simulink model "pmsm_vector_ctrl_osm_2021_07_20"  (R2020a)
settings: Solver=daessc  StartTime=0.0  StopTime=simlength  MaxStep=Ts/10
values from neighbouring files (symbols this model uses):
  dead_time = 0    [init_pmsm_2021_07_20_newDesign.m]    (also in init_pmsm_2021_07_20_oldDesign.m)
  delayINV_modA = 0    [init_pmsm_2021_07_20_newDesign.m]    (also in init_pmsm_2021_07_20_oldDesign.m)
  fPWM_INV = 8e3    (= 8000)    [init_pmsm_2021_07_20_newDesign.m]    (also in init_pmsm_2021_07_20_oldDesign.m)
  Ibez = 550    [init_pmsm_2021_07_20_newDesign.m]    (also in init_pmsm_2021_07_20_oldDesign.m)
  Jm = 1    [init_pmsm_2021_07_20_newDesign.m]    (also in init_pmsm_2021_07_20_oldDesign.m)
  ki = 18    [init_pmsm_2021_07_20_newDesign.m]    (also in init_pmsm_2021_07_20_oldDesign.m)
  kp = 2    [init_pmsm_2021_07_20_newDesign.m]    (also in init_pmsm_2021_07_20_oldDesign.m)
  Ld = 2.77e-3    (= 0.00277)    [init_pmsm_2021_07_20_newDesign.m]    (also in init_pmsm_2021_07_20_oldDesign.m = 0.00267)
  Lq = 3.77e-3    (= 0.00377)    [init_pmsm_2021_07_20_newDesign.m]    (also in init_pmsm_2021_07_20_oldDesign.m = 0.00328)
  number_poles = 8    [init_pmsm_2021_07_20_newDesign.m]    (also in init_pmsm_2021_07_20_oldDesign.m)
  psi_m = 0.5    [init_pmsm_2021_07_20_newDesign.m]    (also in init_pmsm_2021_07_20_oldDesign.m = 0.37)
  simlength = 5    [init_pmsm_2021_07_20_newDesign.m]    (also in init_pmsm_2021_07_20_oldDesign.m)
  Tc = 1e-5    (= 1e-05)    [init_pmsm_2021_07_20_newDesign.m]    (also in init_pmsm_2021_07_20_oldDesign.m)
  Ts = tPWM_INV/2    (= 3.125e-05)    [init_pmsm_2021_07_20_newDesign.m]    (also in init_pmsm_2021_07_20_oldDesign.m)
libraries: nesl_utility x25, fl_lib x23, ee_lib x6, flexshaft_lib x1, pmsm_uvw_lib x1
(part 1 of 2)
settings Model: SimulationMode=accelerator  Creator=dbagn  LastModifiedBy=dbagn
settings SolverCC: ZeroCrossControl=DisableAll  SolverResetMethod=Robust
settings DataIOCC: ReturnWorkspaceOutputs=off

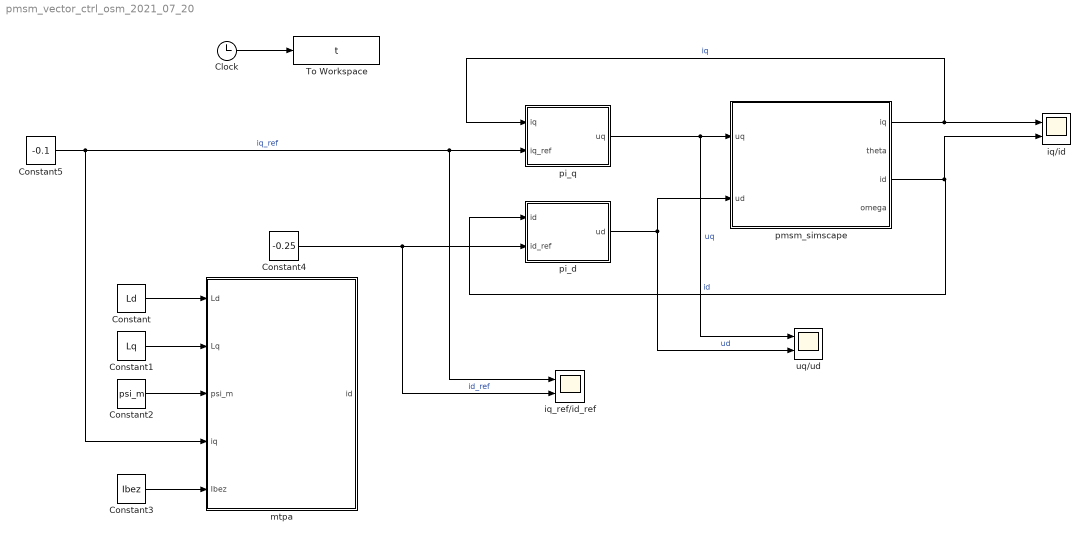
== system pmsm_vector_ctrl_osm_2021_07_20 ==
  Clock : Clock
  Constant : Constant  Value=Ld
  Constant1 : Constant  Value=Lq
  Constant2 : Constant  Value=psi_m
  Constant3 : Constant  Value=Ibez
  Constant4 : Constant  Value=-0.25
  Constant5 : Constant  Value=-0.1
  To Workspace : ToWorkspace  VariableName=t  SampleTime=Tc
      settings: MaxDataPoints=Nc
  iq/id : Scope  NumInputPorts=2
  iq_ref/id_ref : Scope  NumInputPorts=2
  mtpa : MATLAB Function  TreatAsAtomicUnit=on  SystemSampleTime=Ts
  pi_d : Subsystem  mask{kp=kp, ki=ki, ts=Ts, sat_pos=sqrt(3)/2, sat_neg=-sqrt(3)/2}
  pi_q : Subsystem  mask{kp=kp, ki=ki, ts=Ts, sat_pos=sqrt(3)/2, sat_neg=-sqrt(3)/2}
  pmsm_simscape : Subsystem
  uq/ud : Scope  NumInputPorts=2
  wires:
  Clock/1 -> To Workspace/1
  Constant5/1 -> pi_q/2(iq_ref), iq_ref/id_ref/1, mtpa/4(iq)  "iq_ref"
  pmsm_simscape/1(iq) -> iq/id/1, pi_q/1(iq)  "iq"
  pi_q/1(uq) -> uq/ud/1, pmsm_simscape/1(uq)  "uq"
  pi_d/1(ud) -> uq/ud/2, pmsm_simscape/2(ud)  "ud"
  pmsm_simscape/3(id) -> iq/id/2, pi_d/1(id)  "id"
  Constant2/1 -> mtpa/3(psi_m)
  Constant1/1 -> mtpa/2(Lq)
  Constant/1 -> mtpa/1(Ld)
  Constant3/1 -> mtpa/5(Ibez)
  Constant4/1 -> iq_ref/id_ref/2, pi_d/2(id_ref)  "id_ref"

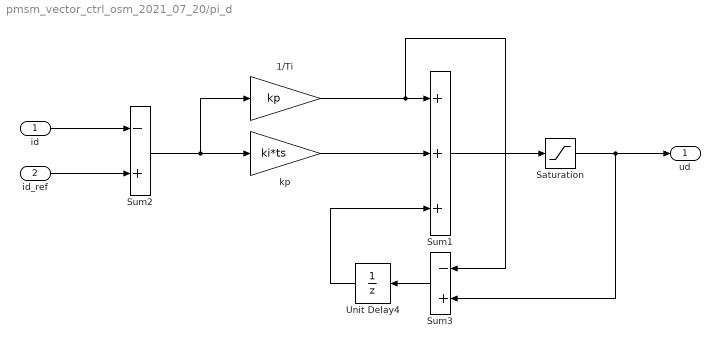
== system pmsm_vector_ctrl_osm_2021_07_20/pi_d ==
  id : Inport
  id_ref : Inport  Port=2
  1/Ti : Gain  Gain=kp  SaturateOnIntegerOverflow=on  OutDataTypeStr=Inherit: Same as input  ParamDataTypeStr=Inherit: Same as input
  Saturation : Saturate  UpperLimit=sat_pos  LowerLimit=sat_neg
  Sum1 : Sum  Inputs=+++  SaturateOnIntegerOverflow=on
  Sum2 : Sum  Inputs=-+  SaturateOnIntegerOverflow=on
  Sum3 : Sum  Inputs=-+  SaturateOnIntegerOverflow=on
  Unit Delay4 : UnitDelay  SampleTime=ts  HasFrameUpgradeWarning=on
  kp : Gain  Gain=ki*ts  SaturateOnIntegerOverflow=on  OutDataTypeStr=Inherit: Same as input  ParamDataTypeStr=Inherit: Same as input
  ud : Outport
  wires:
  Saturation/1 -> Sum3/2, ud/1
  Unit Delay4/1 -> Sum1/3
  Sum1/1 -> Saturation/1
  id/1 -> Sum2/1
  Sum3/1 -> Unit Delay4/1
  1/Ti/1 -> Sum3/1, Sum1/1
  Sum2/1 -> 1/Ti/1, kp/1
  kp/1 -> Sum1/2
  id_ref/1 -> Sum2/2

== system pmsm_vector_ctrl_osm_2021_07_20/pi_q ==
  iq : Inport
  iq_ref : Inport  Port=2
  1/Ti : Gain  Gain=kp  SaturateOnIntegerOverflow=on  OutDataTypeStr=Inherit: Same as input  ParamDataTypeStr=Inherit: Same as input
  Saturation : Saturate  UpperLimit=sat_pos  LowerLimit=sat_neg
  Sum1 : Sum  Inputs=+++  SaturateOnIntegerOverflow=on
  Sum2 : Sum  Inputs=-+  SaturateOnIntegerOverflow=on
  Sum3 : Sum  Inputs=-+  SaturateOnIntegerOverflow=on
  Unit Delay4 : UnitDelay  SampleTime=ts  HasFrameUpgradeWarning=on
  kp : Gain  Gain=ki*ts  SaturateOnIntegerOverflow=on  OutDataTypeStr=Inherit: Same as input  ParamDataTypeStr=Inherit: Same as input
  uq : Outport
  wires:
  iq_ref/1 -> Sum2/2
  kp/1 -> Sum1/2
  Sum2/1 -> kp/1, 1/Ti/1
  1/Ti/1 -> Sum1/1, Sum3/1
  Sum3/1 -> Unit Delay4/1
  iq/1 -> Sum2/1
  Sum1/1 -> Saturation/1
  Unit Delay4/1 -> Sum1/3
  Saturation/1 -> uq/1, Sum3/2

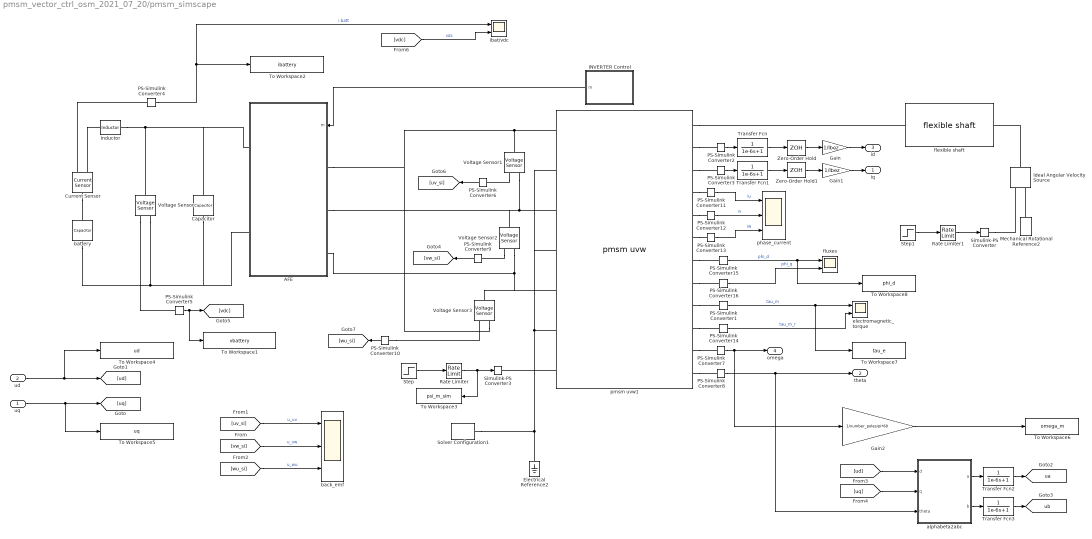
== system pmsm_vector_ctrl_osm_2021_07_20/pmsm_simscape ==
  uq : Inport
  ud : Inport  Port=2
  AFE : Subsystem
  Capacitor : fl_lib/Electrical/Electrical Elements/Capacitor  c=5e-3 F  r=1e-3 Ohm  g=0 1/Ohm  i_specify=off  i_priority=None  i=0 A  i_nominal_specify=off  i_nominal_unit=A  i_nominal_value=1  v_specify=off  v_priority=High  v=350 V  v_nominal_specify=off  v_nominal_unit=V  v_nominal_value=1  vc_specify=on  vc_priority=High  vc=Vdc V  vc_nominal_specify=off  vc_nominal_unit=V  vc_nominal_value=1
  Current Sensor : fl_lib/Electrical/Electrical Sensors/Current Sensor
  Electrical Reference2 : fl_lib/Electrical/Electrical Elements/Electrical Reference
  Gain : Gain  Gain=1/Ibez
  Gain1 : Gain  Gain=1/Ibez
  Gain2 : Gain  Gain=1/number_poles/pi*60
  INVERTER Control : Subsystem
  Ideal Angular Velocity Source : fl_lib/Mechanical/Mechanical Sources/Ideal Angular Velocity Source
  Inductor : fl_lib/Electrical/Electrical Elements/Inductor  l=20e-6 H  r=1e-3 Ohm  g=1e-9 1/Ohm  i_specify=off  i_priority=None  i=0 A  i_nominal_specify=off  i_nominal_unit=A  i_nominal_value=1  v_specify=off  v_priority=None  v=0 V  v_nominal_specify=off  v_nominal_unit=V  v_nominal_value=1  i_L_specify=off  i_L_priority=High  i_L=0 A  i_L_nominal_specify=off  i_L_nominal_unit=A  i_L_nominal_value=1
  Mechanical Rotational Reference2 : fl_lib/Mechanical/Rotational Elements/Mechanical Rotational Reference
  PS-Simulink Converter1 : nesl_utility/PS-Simulink Converter  PhysicalDomain=network_engine_domain  SubClassName=ps_output  LeftPortType=input  RightPortType=output  PseudoPeriodic=off  Frequencies=[]  Unit=N*m  AffineConversion=on
  PS-Simulink Converter{2..4,6,9..10} (6 alike) : nesl_utility/PS-Simulink Converter  PhysicalDomain=network_engine_domain  SubClassName=ps_output  LeftPortType=input  RightPortType=output  PseudoPeriodic=off  Frequencies=[]  Unit=1  AffineConversion=off
  PS-Simulink Converter11 : nesl_utility/PS-Simulink Converter  PhysicalDomain=network_engine_domain  SubClassName=ps_output  LeftPortType=input  RightPortType=output  PseudoPeriodic=off  Frequencies=[]  Unit=A  AffineConversion=on
  PS-Simulink Converter12 : nesl_utility/PS-Simulink Converter  PhysicalDomain=network_engine_domain  SubClassName=ps_output  LeftPortType=input  RightPortType=output  PseudoPeriodic=off  Frequencies=[]  Unit=A  AffineConversion=on
  PS-Simulink Converter13 : nesl_utility/PS-Simulink Converter  PhysicalDomain=network_engine_domain  SubClassName=ps_output  LeftPortType=input  RightPortType=output  PseudoPeriodic=off  Frequencies=[]  Unit=A  AffineConversion=on
  PS-Simulink Converter14 : nesl_utility/PS-Simulink Converter  PhysicalDomain=network_engine_domain  SubClassName=ps_output  LeftPortType=input  RightPortType=output  PseudoPeriodic=off  Frequencies=[]  Unit=N*m  AffineConversion=on
  PS-Simulink Converter15 : nesl_utility/PS-Simulink Converter  PhysicalDomain=network_engine_domain  SubClassName=ps_output  LeftPortType=input  RightPortType=output  PseudoPeriodic=off  Frequencies=[]  Unit=V*s  AffineConversion=on
  PS-Simulink Converter16 : nesl_utility/PS-Simulink Converter  PhysicalDomain=network_engine_domain  SubClassName=ps_output  LeftPortType=input  RightPortType=output  PseudoPeriodic=off  Frequencies=[]  Unit=V*s  AffineConversion=on
  PS-Simulink Converter5 : nesl_utility/PS-Simulink Converter  PhysicalDomain=network_engine_domain  SubClassName=ps_output  LeftPortType=input  RightPortType=output  PseudoPeriodic=off  Frequencies=[]  Unit=V  AffineConversion=on
  PS-Simulink Converter7 : nesl_utility/PS-Simulink Converter  PhysicalDomain=network_engine_domain  SubClassName=ps_output  LeftPortType=input  RightPortType=output  PseudoPeriodic=off  Frequencies=[]  Unit=rad/s  AffineConversion=on
  PS-Simulink Converter8 : nesl_utility/PS-Simulink Converter  PhysicalDomain=network_engine_domain  SubClassName=ps_output  LeftPortType=input  RightPortType=output  PseudoPeriodic=off  Frequencies=[]  Unit=rad  AffineConversion=on
  Rate Limiter : RateLimiter  RisingSlewLimit=0.1  FallingSlewLimit=-0.1  SampleTimeMode=inherited
  Rate Limiter1 : RateLimiter  RisingSlewLimit=3100/2  FallingSlewLimit=-3100/2  SampleTimeMode=inherited
  Simulink-PS Converter : nesl_utility/Simulink-PS Converter  PhysicalDomain=network_engine_domain  SubClassName=ps_input  LeftPortType=input  RightPortType=output  PseudoPeriodic=off  Frequencies=[]  NoiseDistribution=none  NoiseParameters=[]  Unit=rpm  AffineConversion=on  FilteringAndDerivatives=provide  SimscapeFilterOrder=1  InputFilterTimeConstant=0.001  UdotUserProvided=0
  Simulink-PS Converter3 : nesl_utility/Simulink-PS Converter  PhysicalDomain=network_engine_domain  SubClassName=ps_input  LeftPortType=input  RightPortType=output  PseudoPeriodic=off  Frequencies=[]  NoiseDistribution=none  NoiseParameters=[]  Unit=V*s  AffineConversion=off  FilteringAndDerivatives=provide  SimscapeFilterOrder=1  InputFilterTimeConstant=0.001  UdotUserProvided=0
  Solver Configuration1 : nesl_utility/Solver Configuration  PhysicalDomain=network_engine_domain  SubClassName=solver  LeftPortType=input  RightPortType=generic  Tones=[]  Harmonics=[]  SimulateNoise=off  Profile=off  UseLocalSampling=off  EnableSwitchedLinearOptims=on  FrequencyDomain=off  UseCCode=off  RelTol=0.001  AbsTol=1e-06  MinStep=1e-09  ToWorkspace=off  RevertToSquareIcSolve=off  NumHomotopyIterations=100  PhasorMode=off  PhasorModeNumHarmonics=1  DoDC=off  ResidualTolerance=1e-09  UseLocalSolver=on  LocalSolverChoice=NE_BACKWARD_EULER_ADVANCER  LocalSolverSampleTime=Ts/10  DoFixedCost=on  MaxNonlinIter=3  MaxModeIter=2  LinearAlgebra=auto  EquationFormulation=NE_TIME_EF  DelaysMemoryBudget=1024*4  AutomaticFiltering=on  FilteringTimeConstant=Ts  PartitionStorageMethod=AS_NEEDED  PartitionMemoryBudget=1024  PartitionMethod=ROBUST
  Step : Step  Time=simlength/2  Before=psi_m  After=psi_m  SampleTime=0
  Step1 : Step  Time=1e-2  After=3100  SampleTime=0
  To Workspace1 : ToWorkspace  VariableName=vbattery  SampleTime=Tc
      settings: MaxDataPoints=Nc
  To Workspace2 : ToWorkspace  VariableName=ibattery  SampleTime=Tc
      settings: MaxDataPoints=Nc
  To Workspace3 : ToWorkspace  VariableName=psi_m_sim  SampleTime=Tc
      settings: MaxDataPoints=Nc
  To Workspace4 : ToWorkspace  VariableName=ud  SampleTime=Tc
      settings: MaxDataPoints=Nc
  To Workspace5 : ToWorkspace  VariableName=uq  SampleTime=Tc
      settings: MaxDataPoints=Nc
  To Workspace6 : ToWorkspace  VariableName=omega_m  SampleTime=Tc
      settings: MaxDataPoints=Nc
  To Workspace7 : ToWorkspace  VariableName=tau_e  SampleTime=Tc
      settings: MaxDataPoints=Nc
  To Workspace8 : ToWorkspace  VariableName=phi_d  SampleTime=Tc
      settings: MaxDataPoints=Nc
  Transfer Fcn{,1..3} (4 alike) : TransferFcn  Denominator=[1e-6 1]
  Voltage Sensor{,1..3} (4 alike) : fl_lib/Electrical/Electrical Sensors/Voltage Sensor
  Zero-Order Hold : ZeroOrderHold  SampleTime=Ts
  Zero-Order Hold1 : ZeroOrderHold  SampleTime=Ts
  alphabeta2abc : Subsystem
  back_emf : Scope  NumInputPorts=3
  battery : fl_lib/Electrical/Electrical Elements/Capacitor  c=1500 F  r=0.05 Ohm  g=0 1/Ohm  i_specify=off  i_priority=None  i=0 A  i_nominal_specify=off  i_nominal_unit=A  i_nominal_value=1  v_specify=off  v_priority=High  v=350 V  v_nominal_specify=off  v_nominal_unit=V  v_nominal_value=1  vc_specify=on  vc_priority=High  vc=Vdc V  vc_nominal_specify=off  vc_nominal_unit=V  vc_nominal_value=1
  electromagnetic_torque : Scope  NumInputPorts=2
  flexible shaft : flexshaft_lib/flexible shaft  b1=0 N*m/(rad/s)  J1=0.125 kg*m^2  b2=0 N*m/(rad/s)  J2=0.125 kg*m^2  b_theta=1 N*m/(rad/s)  k_theta=1e5 N*m/rad  w_1_specify=off  w_1_priority=None  w_1=0 rad/s  w_1_nominal_specify=off  w_1_nominal_unit=rad/s  w_1_nominal_value=1  w_2_specify=off  w_2_priority=None  w_2=0 rad/s  w_2_nominal_specify=off  w_2_nominal_unit=rad/s  w_2_nominal_value=1  t_1_specify=off  t_1_priority=None  t_1=0 N*m  t_1_nominal_specify=off  t_1_nominal_unit=N*m  t_1_nominal_value=1  t_2_specify=off  t_2_priority=None  t_2=0 N*m  t_2_nominal_specify=off  t_2_nominal_unit=N*m  t_2_nominal_value=1  t_theta_specify=off  t_theta_priority=None  t_theta=0 N*m  t_theta_nominal_specify=off  t_theta_nominal_unit=N*m  t_theta_nominal_value=1
      settings: InternalSimscapePortConfiguration="{\"Bottom\":[],\"Left\":[{\"id\":\"S1\",\"label\":\"S1\",\"type\":\"foundation.mechanical.rotational.rotational\"}],\"Right\":[{\"id\":\"S2\",\"label\":\"S2\",\"type\":\"foundation.mechanical.rotational.rotational\"}],\"Top\":[]}"
  fluxes : Scope  NumInputPorts=2
  ibat/vdc : Scope  NumInputPorts=2
  phase_current : Scope  NumInputPorts=3
  pmsm uvw1 : pmsm_uvw_lib/pmsm uvw  number_poles=number_poles  psi_M=psi_m s*V  Lmu=Lmu H  Ls=Ls H  Lb=Lb H  Rs=Rs Ohm  J=Jm kg*m^2  b=0 N*m/(rad/s)  omega_specify=off  omega_priority=None  omega=0 rad/s  omega_nominal_specify=off  omega_nominal_unit=rad/s  omega_nominal_value=1  theta_specify=off  theta_priority=None  theta=0 rad  theta_nominal_specify=off  theta_nominal_unit=rad  theta_nominal_value=1  iu_specify=off  iu_priority=None  iu=0 A  iu_nominal_specify=off  iu_nominal_unit=A  iu_nominal_value=1  iv_specify=off  iv_priority=None  iv=0 A  iv_nominal_specify=off  iv_nominal_unit=A  iv_nominal_value=1  iw_specify=off  iw_priority=None  iw=0 A  iw_nominal_specify=off  iw_nominal_unit=A  iw_nominal_value=1  id_specify=off  id_priority=None  id=0 A  id_nominal_specify=off  id_nominal_unit=A  id_nominal_value=1  iq_specify=off  iq_priority=None  iq=0 A  iq_nominal_specify=off  iq_nominal_unit=A  iq_nominal_value=1  uv_specify=off  uv_priority=None  uv=0 V  uv_nominal_specify=off  uv_nominal_unit=V  uv_nominal_value=1  uu_specify=off  uu_priority=None  uu=0 V  uu_nominal_specify=off  uu_nominal_unit=V  uu_nominal_value=1  uw_specify=off  uw_priority=None  uw=0 V  uw_nominal_specify=off  uw_nominal_unit=V  uw_nominal_value=1  phi_u_specify=on  phi_u_priority=High  phi_u=psi_m s*V  phi_u_nominal_specify=off  phi_u_nominal_unit=s*V  phi_u_nominal_value=1  phi_v_specify=on  phi_v_priority=High  phi_v=-psi_m/2 s*V  phi_v_nominal_specify=off  phi_v_nominal_unit=s*V  phi_v_nominal_value=1  phi_w_specify=on  phi_w_priority=High  phi_w=-psi_m/2 s*V  phi_w_nominal_specify=off  phi_w_nominal_unit=s*V  phi_w_nominal_value=1  phi_d_specify=off  phi_d_priority=None  phi_d=psi_m s*V  phi_d_nominal_specify=off  phi_d_nominal_unit=s*V  phi_d_nominal_value=1  phi_q_specify=off  phi_q_priority=None  phi_q=0 s*V  phi_q_nominal_specify=off  phi_q_nominal_unit=s*V  phi_q_nominal_value=1  psi_d_specify=off  psi_d_priority=None  psi_d=0 s*V  psi_d_nominal_specify=off  psi_d_nominal_unit=s*V  psi_d_nominal_value=1  psi_q_specify=off  psi_q_priority=None  psi_q=0 s*V  psi_q_nominal_specify=off  psi_q_nominal_unit=s*V  psi_q_nominal_value=1  tau_l_specify=off  tau_l_priority=None  tau_l=0 N*m  tau_l_nominal_specify=off  tau_l_nominal_unit=N*m  tau_l_nominal_value=1  tau_m_specify=off  tau_m_priority=None  tau_m=0 N*m  tau_m_nominal_specify=off  tau_m_nominal_unit=N*m  tau_m_nominal_value=1  tau_m_r_specify=off  tau_m_r_priority=None  tau_m_r=0 N*m  tau_m_r_nominal_specify=off  tau_m_r_nominal_unit=N*m  tau_m_r_nominal_value=1
      settings: InternalSimscapePortConfiguration="{\"Bottom\":[],\"Left\":[{\"id\":\"uu_p\",\"label\":\"_uu+_\",\"type\":\"foundation.electrical.electrical\"},{\"id\":\"uu_n\",\"label\":\"_uu-_\",\"type\":\"foundation.electrical.electrical\"},{\"id\":\"uv_p\",\"label\":\"_uv+_\",\"type\":\"foundation.electrical.electrical\"},{\"id\":\"uv_n\",\"label\":\"_uv-_\",\"type\":\"foundation.electrical.electrical\"},{\"id\":\"uw_p\",\"label\":\"_uw+_\",\"type\":\"foundation.electrical.electrical\"},{\"id\":\"uw_n\",\"label\":\"_uw-_\",\"type\":\"foundation.electrical.electrical\"},{\"id\":\"psi_m\",\"label\":\"_psi_m_\",\"type\":\"input\"}],\"Right\":[{\"id\":\"S\",\"label\":\"_S_\",\"type\":\"foundation.mechanical.rotational.rotational\"},{\"id\":\"id_out\",\"label\":\"_id_\",\"type\":\"output\"},{\"id\":\"iq_out\",\"label\":\"_iq_\",\"type\":\"output\"},{\"id\":\"iu_out\",\"label\":\"_iu_\",\"type\":\"output\"},{\"id\":\"iv_out\",\"label\":\"_iv_\",\"type\":\"output\"},{\"id\":\"iw_out\",\"label\":\"_iw_\",\"type\":\"output\"},{\"id\":\"phi_d_out\",\"label\":\"_phi_d_\",\"type\":\"output\"},{\"id\":\"phi_q_out\",\"label\":\"_phi_q\",\"type\":\"output\"},{\"id\":\"tau_out\",\"label\":\"_torque_\",\"type\":\"output\"},{\"id\":\"tau_out_r\",\"label\":\"_torque_r_\",\"type\":\"output\"},{\"id\":\"omega_out\",\"label\":\"_omega_elec_\",\"type\":\"output\"},{\"id\":\"theta_out\",\"label\":\"_theta_elec_\",\"type\":\"output\"}],\"Top\":[]}"
  iq : Outport
  theta : Outport  Port=2
  id : Outport  Port=3
  omega : Outport  Port=4
  tag scope: ua=global, ub=global
  wires:
  PS-Simulink Converter2/1 -> Transfer Fcn/1
  PS-Simulink Converter3/1 -> Transfer Fcn1/1
  [ud] -> alphabeta2abc/1(d)
  [uq] -> alphabeta2abc/2(q)
  alphabeta2abc/1(a) -> Transfer Fcn2/1
  alphabeta2abc/2(b) -> Transfer Fcn3/1
  Zero-Order Hold/1 -> Gain/1
  Zero-Order Hold1/1 -> Gain1/1
  Rate Limiter/1 -> To Workspace3/1, Simulink-PS Converter3/1
  Step/1 -> Rate Limiter/1
  Transfer Fcn/1 -> Zero-Order Hold/1
  Transfer Fcn1/1 -> Zero-Order Hold1/1
  PS-Simulink Converter8/1 -> alphabeta2abc/3(theta), theta/1
  ud/1 -> To Workspace4/1, [ud]
  uq/1 -> To Workspace5/1, [uq]
  Transfer Fcn2/1 -> [ua]
  Transfer Fcn3/1 -> [ub]
  Gain/1 -> id/1
  Gain1/1 -> iq/1
  PS-Simulink Converter1/1 -> To Workspace7/1, electromagnetic_torque/1  "tau_m"
  PS-Simulink Converter4/1 -> ibat/vdc/1, To Workspace2/1  "i batt"
  PS-Simulink Converter6/1 -> [uv_si]
  PS-Simulink Converter7/1 -> Gain2/1, omega/1
  Step1/1 -> Rate Limiter1/1
  Rate Limiter1/1 -> Simulink-PS Converter/1
  PS-Simulink Converter12/1 -> phase_current/2  "iv"
  PS-Simulink Converter11/1 -> phase_current/1  "iu"
  PS-Simulink Converter13/1 -> phase_current/3  "iw"
  [wu_si] -> back_emf/3  "u_wu"
  [vw_si] -> back_emf/2  "u_vw"
  [uv_si] -> back_emf/1  "u_uv"
  PS-Simulink Converter9/1 -> [vw_si]
  PS-Simulink Converter10/1 -> [wu_si]
  [vdc] -> ibat/vdc/2  "vdc"
  INVERTER Control/1(m) -> AFE/1(m)
  PS-Simulink Converter14/1 -> electromagnetic_torque/2  "tau_m_r"
  PS-Simulink Converter15/1 -> To Workspace8/1, fluxes/1  "phi_d"
  PS-Simulink Converter16/1 -> fluxes/2  "phi_q"
  PS-Simulink Converter5/1 -> To Workspace1/1, [vdc]
  Gain2/1 -> To Workspace6/1
  connections:
  Voltage Sensor1/RConn2 -- pmsm uvw1/LConn3 -- Voltage Sensor2/LConn1 -- AFE/LConn2
  Voltage Sensor1/LConn1 -- AFE/LConn1 -- Voltage Sensor3/RConn2 -- pmsm uvw1/LConn1
  Electrical Reference2/LConn1 -- Solver Configuration1/RConn1 -- pmsm uvw1/LConn6 -- pmsm uvw1/LConn2 -- pmsm uvw1/LConn4
  pmsm uvw1/LConn7 -- Simulink-PS Converter3/RConn1
  pmsm uvw1/RConn2 -- PS-Simulink Converter2/LConn1
  pmsm uvw1/RConn3 -- PS-Simulink Converter3/LConn1
  pmsm uvw1/RConn9 -- PS-Simulink Converter1/LConn1
  Voltage Sensor1/RConn1 -- PS-Simulink Converter6/LConn1
  AFE/LConn3 -- pmsm uvw1/LConn5 -- Voltage Sensor3/LConn1 -- Voltage Sensor2/RConn2
  Ideal Angular Velocity Source/LConn1 -- flexible shaft/RConn1
  Simulink-PS Converter/RConn1 -- Ideal Angular Velocity Source/RConn1
  Mechanical Rotational Reference2/LConn1 -- Ideal Angular Velocity Source/RConn2
  pmsm uvw1/RConn1 -- flexible shaft/LConn1
  Voltage Sensor/RConn2 -- battery/RConn1 -- AFE/RConn2 -- Capacitor/RConn1
  Current Sensor/LConn1 -- battery/LConn1
  Voltage Sensor/RConn1 -- PS-Simulink Converter5/LConn1
  Current Sensor/RConn1 -- PS-Simulink Converter4/LConn1
  Voltage Sensor/LConn1 -- Capacitor/LConn1 -- AFE/RConn1 -- Inductor/RConn1
  pmsm uvw1/RConn6 -- PS-Simulink Converter13/LConn1
  pmsm uvw1/RConn4 -- PS-Simulink Converter11/LConn1
  pmsm uvw1/RConn5 -- PS-Simulink Converter12/LConn1
  Voltage Sensor2/RConn1 -- PS-Simulink Converter9/LConn1
  PS-Simulink Converter10/LConn1 -- Voltage Sensor3/RConn1
  Current Sensor/RConn2 -- Inductor/LConn1
  pmsm uvw1/RConn11 -- PS-Simulink Converter7/LConn1
  pmsm uvw1/RConn12 -- PS-Simulink Converter8/LConn1
  pmsm uvw1/RConn10 -- PS-Simulink Converter14/LConn1
  pmsm uvw1/RConn7 -- PS-Simulink Converter15/LConn1
  pmsm uvw1/RConn8 -- PS-Simulink Converter16/LConn1

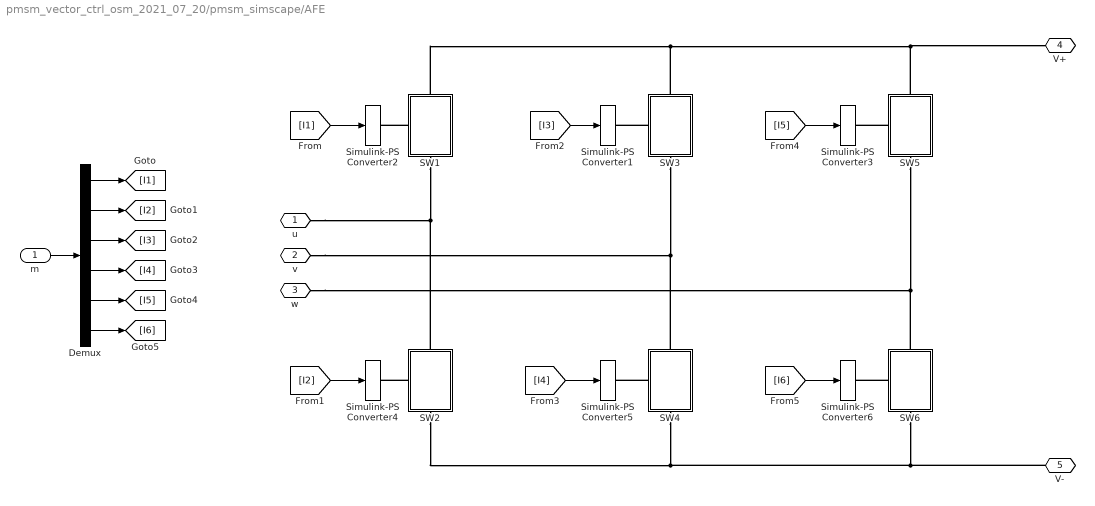
== system pmsm_vector_ctrl_osm_2021_07_20/pmsm_simscape/AFE ==
  m : Inport
  Demux : Demux  Outputs=6
  SW1 : Subsystem
      settings: PortSchema="{\"entries\":[{\"content\":{\"sides\":[{\"content\":{\"connectorIds\":[\"LConn1\"]},\"type\":\"ConnectorPlacement.EquallySpacedRectSide\",\"uuid\":\"ebeefb4b-0693-4cf6-af95-ed1786d6fcd3\"},{\"content\":{\"connectorIds\":[],\"side\":\"RIGHT\"},\"type\":\"ConnectorPlacement.EquallySpacedRectSide\",\"uuid\":\"b6a4070d-be39-4125-92ef-a5915edd47f8\"},{\"content\":{\"connectorIds\":[\"LConn2\"],\"side\":\"TOP\"},\"type\":\"ConnectorPlacement.EquallySpacedRectSide\",\"uuid\":\"2e4d4478-0972-498e-853c-615c31998c86\"},{\"content\":{\"connectorIds\":[\"RConn1\"],\"side\":\"BOTTOM\"},\"type\":\"ConnectorPlacement.EquallySpacedRectSide\",\"uuid\":\"9f2b7d21-f53a-43c3-94e3-6e1994c38f8b\"}]},\"type\":\"ConnectorPlacement.EquallySpacedConnector\",\"uuid\":\"0cb5dd33-96f4-4c61-9960-19c566731d51\"}],\"packageUris\":[\"http://schema.mathworks.com/mf0/Connector/19700101\"],\"version\":\"1.0\"}"
  SW2 : Subsystem
      settings: PortSchema="{\"entries\":[{\"content\":{\"sides\":[{\"content\":{\"connectorIds\":[\"LConn1\"]},\"type\":\"ConnectorPlacement.EquallySpacedRectSide\",\"uuid\":\"ebeefb4b-0693-4cf6-af95-ed1786d6fcd3\"},{\"content\":{\"connectorIds\":[],\"side\":\"RIGHT\"},\"type\":\"ConnectorPlacement.EquallySpacedRectSide\",\"uuid\":\"b6a4070d-be39-4125-92ef-a5915edd47f8\"},{\"content\":{\"connectorIds\":[\"LConn2\"],\"side\":\"TOP\"},\"type\":\"ConnectorPlacement.EquallySpacedRectSide\",\"uuid\":\"2e4d4478-0972-498e-853c-615c31998c86\"},{\"content\":{\"connectorIds\":[\"RConn1\"],\"side\":\"BOTTOM\"},\"type\":\"ConnectorPlacement.EquallySpacedRectSide\",\"uuid\":\"9f2b7d21-f53a-43c3-94e3-6e1994c38f8b\"}]},\"type\":\"ConnectorPlacement.EquallySpacedConnector\",\"uuid\":\"0cb5dd33-96f4-4c61-9960-19c566731d51\"}],\"packageUris\":[\"http://schema.mathworks.com/mf0/Connector/19700101\"],\"version\":\"1.0\"}"
  SW3 : Subsystem
      settings: PortSchema="{\"entries\":[{\"content\":{\"sides\":[{\"content\":{\"connectorIds\":[\"LConn1\"]},\"type\":\"ConnectorPlacement.EquallySpacedRectSide\",\"uuid\":\"ebeefb4b-0693-4cf6-af95-ed1786d6fcd3\"},{\"content\":{\"connectorIds\":[],\"side\":\"RIGHT\"},\"type\":\"ConnectorPlacement.EquallySpacedRectSide\",\"uuid\":\"b6a4070d-be39-4125-92ef-a5915edd47f8\"},{\"content\":{\"connectorIds\":[\"LConn2\"],\"side\":\"TOP\"},\"type\":\"ConnectorPlacement.EquallySpacedRectSide\",\"uuid\":\"2e4d4478-0972-498e-853c-615c31998c86\"},{\"content\":{\"connectorIds\":[\"RConn1\"],\"side\":\"BOTTOM\"},\"type\":\"ConnectorPlacement.EquallySpacedRectSide\",\"uuid\":\"9f2b7d21-f53a-43c3-94e3-6e1994c38f8b\"}]},\"type\":\"ConnectorPlacement.EquallySpacedConnector\",\"uuid\":\"0cb5dd33-96f4-4c61-9960-19c566731d51\"}],\"packageUris\":[\"http://schema.mathworks.com/mf0/Connector/19700101\"],\"version\":\"1.0\"}"
  SW4 : Subsystem
      settings: PortSchema="{\"entries\":[{\"content\":{\"sides\":[{\"content\":{\"connectorIds\":[\"LConn1\"]},\"type\":\"ConnectorPlacement.EquallySpacedRectSide\",\"uuid\":\"ebeefb4b-0693-4cf6-af95-ed1786d6fcd3\"},{\"content\":{\"connectorIds\":[],\"side\":\"RIGHT\"},\"type\":\"ConnectorPlacement.EquallySpacedRectSide\",\"uuid\":\"b6a4070d-be39-4125-92ef-a5915edd47f8\"},{\"content\":{\"connectorIds\":[\"LConn2\"],\"side\":\"TOP\"},\"type\":\"ConnectorPlacement.EquallySpacedRectSide\",\"uuid\":\"2e4d4478-0972-498e-853c-615c31998c86\"},{\"content\":{\"connectorIds\":[\"RConn1\"],\"side\":\"BOTTOM\"},\"type\":\"ConnectorPlacement.EquallySpacedRectSide\",\"uuid\":\"9f2b7d21-f53a-43c3-94e3-6e1994c38f8b\"}]},\"type\":\"ConnectorPlacement.EquallySpacedConnector\",\"uuid\":\"0cb5dd33-96f4-4c61-9960-19c566731d51\"}],\"packageUris\":[\"http://schema.mathworks.com/mf0/Connector/19700101\"],\"version\":\"1.0\"}"
  SW5 : Subsystem
      settings: PortSchema="{\"entries\":[{\"content\":{\"sides\":[{\"content\":{\"connectorIds\":[\"LConn1\"]},\"type\":\"ConnectorPlacement.EquallySpacedRectSide\",\"uuid\":\"ebeefb4b-0693-4cf6-af95-ed1786d6fcd3\"},{\"content\":{\"connectorIds\":[],\"side\":\"RIGHT\"},\"type\":\"ConnectorPlacement.EquallySpacedRectSide\",\"uuid\":\"b6a4070d-be39-4125-92ef-a5915edd47f8\"},{\"content\":{\"connectorIds\":[\"LConn2\"],\"side\":\"TOP\"},\"type\":\"ConnectorPlacement.EquallySpacedRectSide\",\"uuid\":\"2e4d4478-0972-498e-853c-615c31998c86\"},{\"content\":{\"connectorIds\":[\"RConn1\"],\"side\":\"BOTTOM\"},\"type\":\"ConnectorPlacement.EquallySpacedRectSide\",\"uuid\":\"9f2b7d21-f53a-43c3-94e3-6e1994c38f8b\"}]},\"type\":\"ConnectorPlacement.EquallySpacedConnector\",\"uuid\":\"0cb5dd33-96f4-4c61-9960-19c566731d51\"}],\"packageUris\":[\"http://schema.mathworks.com/mf0/Connector/19700101\"],\"version\":\"1.0\"}"
  SW6 : Subsystem
      settings: PortSchema="{\"entries\":[{\"content\":{\"sides\":[{\"content\":{\"connectorIds\":[\"LConn1\"]},\"type\":\"ConnectorPlacement.EquallySpacedRectSide\",\"uuid\":\"ebeefb4b-0693-4cf6-af95-ed1786d6fcd3\"},{\"content\":{\"connectorIds\":[],\"side\":\"RIGHT\"},\"type\":\"ConnectorPlacement.EquallySpacedRectSide\",\"uuid\":\"b6a4070d-be39-4125-92ef-a5915edd47f8\"},{\"content\":{\"connectorIds\":[\"LConn2\"],\"side\":\"TOP\"},\"type\":\"ConnectorPlacement.EquallySpacedRectSide\",\"uuid\":\"2e4d4478-0972-498e-853c-615c31998c86\"},{\"content\":{\"connectorIds\":[\"RConn1\"],\"side\":\"BOTTOM\"},\"type\":\"ConnectorPlacement.EquallySpacedRectSide\",\"uuid\":\"9f2b7d21-f53a-43c3-94e3-6e1994c38f8b\"}]},\"type\":\"ConnectorPlacement.EquallySpacedConnector\",\"uuid\":\"0cb5dd33-96f4-4c61-9960-19c566731d51\"}],\"packageUris\":[\"http://schema.mathworks.com/mf0/Connector/19700101\"],\"version\":\"1.0\"}"
  Simulink-PS Converter{1..6} (6 alike) : nesl_utility/Simulink-PS Converter  PhysicalDomain=network_engine_domain  SubClassName=ps_input  LeftPortType=input  RightPortType=output  PseudoPeriodic=off  Frequencies=[]  NoiseDistribution=none  NoiseParameters=[]  Unit=V  AffineConversion=off  FilteringAndDerivatives=zero  SimscapeFilterOrder=2  InputFilterTimeConstant=Tc  UdotUserProvided=2
  u : PMIOPort  Side=Left
  v : PMIOPort  Port=2  Side=Left
  w : PMIOPort  Port=3  Side=Left
  V+ : PMIOPort  Port=4  Side=Right
  V- : PMIOPort  Port=5  Side=Right
  wires:
  m/1 -> Demux/1
  Demux/1 -> [I1]
  Demux/2 -> [I2]
  Demux/3 -> [I3]
  Demux/4 -> [I4]
  Demux/5 -> [I5]
  Demux/6 -> [I6]
  [I1] -> Simulink-PS Converter2/1
  [I3] -> Simulink-PS Converter1/1
  [I5] -> Simulink-PS Converter3/1
  [I2] -> Simulink-PS Converter4/1
  [I6] -> Simulink-PS Converter6/1
  [I4] -> Simulink-PS Converter5/1
  connections:
  u/RConn1 -- SW2/LConn2 -- SW1/RConn1
  v/RConn1 -- SW4/LConn2 -- SW3/RConn1
  w/RConn1 -- SW6/LConn2 -- SW5/RConn1
  SW1/LConn1 -- Simulink-PS Converter2/RConn1
  SW1/LConn2 -- SW3/LConn2 -- SW5/LConn2 -- V+/RConn1
  V-/RConn1 -- SW6/RConn1 -- SW4/RConn1 -- SW2/RConn1
  SW3/LConn1 -- Simulink-PS Converter1/RConn1
  SW5/LConn1 -- Simulink-PS Converter3/RConn1
  SW6/LConn1 -- Simulink-PS Converter6/RConn1
  SW4/LConn1 -- Simulink-PS Converter5/RConn1
  SW2/LConn1 -- Simulink-PS Converter4/RConn1

== system pmsm_vector_ctrl_osm_2021_07_20/pmsm_simscape/INVERTER Control ==
  Bus Creator1 : BusCreator  Inputs=2
  PWM generator1 : Subsystem
  Product : Product
  Step : Step  Time=simlength*4/5  Before=1  After=0  SampleTime=0
  m : Outport  VectorParamsAs1DForOutWhenUnconnected=off
  wires:
  [ub] -> Bus Creator1/2
  Bus Creator1/1 -> PWM generator1/1(uab)
  [ua] -> Bus Creator1/1
  PWM generator1/1(m) -> Product/2
  Product/1 -> m/1
  Step/1 -> Product/1

== system pmsm_vector_ctrl_osm_2021_07_20/pmsm_simscape/alphabeta2abc ==
  d : Inport
  q : Inport  Port=2
  theta : Inport  Port=3
  alphabeta2xieta : Subsystem
  a : Outport  VectorParamsAs1DForOutWhenUnconnected=off
  b : Outport  Port=2  VectorParamsAs1DForOutWhenUnconnected=off
  wires:
  theta/1 -> alphabeta2xieta/3(theta)
  d/1 -> alphabeta2xieta/1(d)
  q/1 -> alphabeta2xieta/2(q)
  alphabeta2xieta/1(alpha) -> a/1
  alphabeta2xieta/2(beta) -> b/1

== system pmsm_vector_ctrl_osm_2021_07_20/pmsm_simscape/AFE/SW1 ==
  Diode : ee_lib/Semiconductors & Converters/Diode  ModelType=ee.enum.diode.modelType.pwl  Vf=1.9 V  Ron=Ron Ohm  Goff=1e-8 S  prmExp=ee.enum.diode.expParam.useTwo  I12=[.0137, .545] A  V12=[.6, .7] V  IS=1e-12 A  ec=1  I1=0.0137 A  V1=0.6 V  RS=0 Ohm  Tmeas=25 degC  N_series=1  N_parallel=1  Rz=0.3 Ohm  BV=inf V  C_param=ee.enum.diode.capParam.fixed  CJ=5 pF  CJ0=5 pF  VJ=1 V  Mgrad=0.5  Vvec=[.1, 10, 100] V  Cvec=[3.5, 1, .4] pF  FC=0.5  Q_param=ee.enum.diode.recoveryParam.off  iRM=-7.15 A  iF=4 A  didt=-750 A/us  trr_factor=3  trr=115 ns  Qrr=1500 s*uA  TT=50 ns  tau=100 ns  T_param=ee.enum.diode.temperatureParam.off  IS_T2=1.25e-7 A  I1_T2=0.245 A  V1_T2=0.5 V  Tmeas2=125 degC  EG_param=ee.enum.diode.egapParam.material_si  EG=1.11 eV  XTI_param=ee.enum.diode.xtiParam.pn  XTI=3  dBVdT=0 V/K  Tdevice=25 degC  i_specify=off  i_priority=None  i=0 A  i_nominal_specify=off  i_nominal_unit=A  i_nominal_value=1  v_specify=off  v_priority=None  v=0 V  v_nominal_specify=off  v_nominal_unit=V  v_nominal_value=1  i_capacitor_specify=off  i_capacitor_priority=None  i_capacitor=0 A  i_capacitor_nominal_specify=off  i_capacitor_nominal_unit=A  i_capacitor_nominal_value=1  v_capacitor_specify=off  v_capacitor_priority=None  v_capacitor=0 V  v_capacitor_nominal_specify=off  v_capacitor_nominal_unit=V  v_capacitor_nominal_value=1  power_dissipated_specify=off  power_dissipated_priority=None  power_dissipated=0 W  power_dissipated_nominal_specify=off  power_dissipated_nominal_unit=W  power_dissipated_nominal_value=1  thermal_network_parameterization=ee.enum.thermalNetworkTopology.cauer  Rth=[0, 10] K/W  Rth_Foster=[4, 6] K/W  thermal_mass_parameterization=ee.enum.thermalNetwork.timeconstant  thermal_mass=[0, 1] J/K  thermal_mass_Foster=[1.5, 3] J/K  thermal_time_constant=[0, 10] s  thermal_time_constant_Foster=[6, 18] s  thermal_mass_initial_temperatures=[25, 25] degC
  Diode1 : fl_lib/Electrical/Electrical Elements/Diode  Vf=0.6 V  Ron=Ron Ohm  Goff=1e-8 1/Ohm  i_specify=off  i_priority=None  i=0 A  i_nominal_specify=off  i_nominal_unit=A  i_nominal_value=1  v_specify=off  v_priority=None  v=0 V  v_nominal_specify=off  v_nominal_unit=V  v_nominal_value=1
  Switch : fl_lib/Electrical/Electrical Elements/Switch  R_closed=Ron Ohm  G_open=1e-8 1/Ohm  Threshold=0.5  i_specify=off  i_priority=None  i=0 A  i_nominal_specify=off  i_nominal_unit=A  i_nominal_value=1  v_specify=off  v_priority=None  v=0 V  v_nominal_specify=off  v_nominal_unit=V  v_nominal_value=1
  G : PMIOPort  Side=Left
  D : PMIOPort  Port=2  Side=Left
  S : PMIOPort  Port=3  Side=Right
  connections:
  Diode/LConn1 -- S/RConn1 -- Switch/RConn2
  Diode/RConn1 -- Switch/LConn1 -- D/RConn1
  G/RConn1 -- Switch/RConn1

== system pmsm_vector_ctrl_osm_2021_07_20/pmsm_simscape/AFE/SW2 ==
  Diode : ee_lib/Semiconductors & Converters/Diode  ModelType=ee.enum.diode.modelType.pwl  Vf=1.9 V  Ron=Ron Ohm  Goff=1e-8 S  prmExp=ee.enum.diode.expParam.useTwo  I12=[.0137, .545] A  V12=[.6, .7] V  IS=1e-12 A  ec=1  I1=0.0137 A  V1=0.6 V  RS=0 Ohm  Tmeas=25 degC  N_series=1  N_parallel=1  Rz=0.3 Ohm  BV=inf V  C_param=ee.enum.diode.capParam.fixed  CJ=5 pF  CJ0=5 pF  VJ=1 V  Mgrad=0.5  Vvec=[.1, 10, 100] V  Cvec=[3.5, 1, .4] pF  FC=0.5  Q_param=ee.enum.diode.recoveryParam.off  iRM=-7.15 A  iF=4 A  didt=-750 A/us  trr_factor=3  trr=115 ns  Qrr=1500 s*uA  TT=50 ns  tau=100 ns  T_param=ee.enum.diode.temperatureParam.off  IS_T2=1.25e-7 A  I1_T2=0.245 A  V1_T2=0.5 V  Tmeas2=125 degC  EG_param=ee.enum.diode.egapParam.material_si  EG=1.11 eV  XTI_param=ee.enum.diode.xtiParam.pn  XTI=3  dBVdT=0 V/K  Tdevice=25 degC  i_specify=off  i_priority=None  i=0 A  i_nominal_specify=off  i_nominal_unit=A  i_nominal_value=1  v_specify=off  v_priority=None  v=0 V  v_nominal_specify=off  v_nominal_unit=V  v_nominal_value=1  i_capacitor_specify=off  i_capacitor_priority=None  i_capacitor=0 A  i_capacitor_nominal_specify=off  i_capacitor_nominal_unit=A  i_capacitor_nominal_value=1  v_capacitor_specify=off  v_capacitor_priority=None  v_capacitor=0 V  v_capacitor_nominal_specify=off  v_capacitor_nominal_unit=V  v_capacitor_nominal_value=1  power_dissipated_specify=off  power_dissipated_priority=None  power_dissipated=0 W  power_dissipated_nominal_specify=off  power_dissipated_nominal_unit=W  power_dissipated_nominal_value=1  thermal_network_parameterization=ee.enum.thermalNetworkTopology.cauer  Rth=[0, 10] K/W  Rth_Foster=[4, 6] K/W  thermal_mass_parameterization=ee.enum.thermalNetwork.timeconstant  thermal_mass=[0, 1] J/K  thermal_mass_Foster=[1.5, 3] J/K  thermal_time_constant=[0, 10] s  thermal_time_constant_Foster=[6, 18] s  thermal_mass_initial_temperatures=[25, 25] degC
  Diode1 : fl_lib/Electrical/Electrical Elements/Diode  Vf=0.6 V  Ron=Ron Ohm  Goff=1e-8 1/Ohm  i_specify=off  i_priority=None  i=0 A  i_nominal_specify=off  i_nominal_unit=A  i_nominal_value=1  v_specify=off  v_priority=None  v=0 V  v_nominal_specify=off  v_nominal_unit=V  v_nominal_value=1
  Switch : fl_lib/Electrical/Electrical Elements/Switch  R_closed=Ron Ohm  G_open=1e-8 1/Ohm  Threshold=0.5  i_specify=off  i_priority=None  i=0 A  i_nominal_specify=off  i_nominal_unit=A  i_nominal_value=1  v_specify=off  v_priority=None  v=0 V  v_nominal_specify=off  v_nominal_unit=V  v_nominal_value=1
  G : PMIOPort  Side=Left
  D : PMIOPort  Port=2  Side=Left
  S : PMIOPort  Port=3  Side=Right
  connections:
  G/RConn1 -- Switch/RConn1
  Switch/LConn1 -- D/RConn1 -- Diode/RConn1
  S/RConn1 -- Switch/RConn2 -- Diode/LConn1

== system pmsm_vector_ctrl_osm_2021_07_20/pmsm_simscape/AFE/SW3 ==
  Diode : ee_lib/Semiconductors & Converters/Diode  ModelType=ee.enum.diode.modelType.pwl  Vf=1.9 V  Ron=Ron Ohm  Goff=1e-8 S  prmExp=ee.enum.diode.expParam.useTwo  I12=[.0137, .545] A  V12=[.6, .7] V  IS=1e-12 A  ec=1  I1=0.0137 A  V1=0.6 V  RS=0 Ohm  Tmeas=25 degC  N_series=1  N_parallel=1  Rz=0.3 Ohm  BV=inf V  C_param=ee.enum.diode.capParam.fixed  CJ=5 pF  CJ0=5 pF  VJ=1 V  Mgrad=0.5  Vvec=[.1, 10, 100] V  Cvec=[3.5, 1, .4] pF  FC=0.5  Q_param=ee.enum.diode.recoveryParam.off  iRM=-7.15 A  iF=4 A  didt=-750 A/us  trr_factor=3  trr=115 ns  Qrr=1500 s*uA  TT=50 ns  tau=100 ns  T_param=ee.enum.diode.temperatureParam.off  IS_T2=1.25e-7 A  I1_T2=0.245 A  V1_T2=0.5 V  Tmeas2=125 degC  EG_param=ee.enum.diode.egapParam.material_si  EG=1.11 eV  XTI_param=ee.enum.diode.xtiParam.pn  XTI=3  dBVdT=0 V/K  Tdevice=25 degC  i_specify=off  i_priority=None  i=0 A  i_nominal_specify=off  i_nominal_unit=A  i_nominal_value=1  v_specify=off  v_priority=None  v=0 V  v_nominal_specify=off  v_nominal_unit=V  v_nominal_value=1  i_capacitor_specify=off  i_capacitor_priority=None  i_capacitor=0 A  i_capacitor_nominal_specify=off  i_capacitor_nominal_unit=A  i_capacitor_nominal_value=1  v_capacitor_specify=off  v_capacitor_priority=None  v_capacitor=0 V  v_capacitor_nominal_specify=off  v_capacitor_nominal_unit=V  v_capacitor_nominal_value=1  power_dissipated_specify=off  power_dissipated_priority=None  power_dissipated=0 W  power_dissipated_nominal_specify=off  power_dissipated_nominal_unit=W  power_dissipated_nominal_value=1  thermal_network_parameterization=ee.enum.thermalNetworkTopology.cauer  Rth=[0, 10] K/W  Rth_Foster=[4, 6] K/W  thermal_mass_parameterization=ee.enum.thermalNetwork.timeconstant  thermal_mass=[0, 1] J/K  thermal_mass_Foster=[1.5, 3] J/K  thermal_time_constant=[0, 10] s  thermal_time_constant_Foster=[6, 18] s  thermal_mass_initial_temperatures=[25, 25] degC
  Diode1 : fl_lib/Electrical/Electrical Elements/Diode  Vf=0.6 V  Ron=Ron Ohm  Goff=1e-8 1/Ohm  i_specify=off  i_priority=None  i=0 A  i_nominal_specify=off  i_nominal_unit=A  i_nominal_value=1  v_specify=off  v_priority=None  v=0 V  v_nominal_specify=off  v_nominal_unit=V  v_nominal_value=1
  Switch : fl_lib/Electrical/Electrical Elements/Switch  R_closed=Ron Ohm  G_open=1e-8 1/Ohm  Threshold=0.5  i_specify=off  i_priority=None  i=0 A  i_nominal_specify=off  i_nominal_unit=A  i_nominal_value=1  v_specify=off  v_priority=None  v=0 V  v_nominal_specify=off  v_nominal_unit=V  v_nominal_value=1
  G : PMIOPort  Side=Left
  D : PMIOPort  Port=2  Side=Left
  S : PMIOPort  Port=3  Side=Right
  connections:
  Diode/LConn1 -- Switch/RConn2 -- S/RConn1
  Diode/RConn1 -- D/RConn1 -- Switch/LConn1
  G/RConn1 -- Switch/RConn1

== system pmsm_vector_ctrl_osm_2021_07_20/pmsm_simscape/AFE/SW4 ==
  Diode : ee_lib/Semiconductors & Converters/Diode  ModelType=ee.enum.diode.modelType.pwl  Vf=1.9 V  Ron=Ron Ohm  Goff=1e-8 S  prmExp=ee.enum.diode.expParam.useTwo  I12=[.0137, .545] A  V12=[.6, .7] V  IS=1e-12 A  ec=1  I1=0.0137 A  V1=0.6 V  RS=0 Ohm  Tmeas=25 degC  N_series=1  N_parallel=1  Rz=0.3 Ohm  BV=inf V  C_param=ee.enum.diode.capParam.fixed  CJ=5 pF  CJ0=5 pF  VJ=1 V  Mgrad=0.5  Vvec=[.1, 10, 100] V  Cvec=[3.5, 1, .4] pF  FC=0.5  Q_param=ee.enum.diode.recoveryParam.off  iRM=-7.15 A  iF=4 A  didt=-750 A/us  trr_factor=3  trr=115 ns  Qrr=1500 s*uA  TT=50 ns  tau=100 ns  T_param=ee.enum.diode.temperatureParam.off  IS_T2=1.25e-7 A  I1_T2=0.245 A  V1_T2=0.5 V  Tmeas2=125 degC  EG_param=ee.enum.diode.egapParam.material_si  EG=1.11 eV  XTI_param=ee.enum.diode.xtiParam.pn  XTI=3  dBVdT=0 V/K  Tdevice=25 degC  i_specify=off  i_priority=None  i=0 A  i_nominal_specify=off  i_nominal_unit=A  i_nominal_value=1  v_specify=off  v_priority=None  v=0 V  v_nominal_specify=off  v_nominal_unit=V  v_nominal_value=1  i_capacitor_specify=off  i_capacitor_priority=None  i_capacitor=0 A  i_capacitor_nominal_specify=off  i_capacitor_nominal_unit=A  i_capacitor_nominal_value=1  v_capacitor_specify=off  v_capacitor_priority=None  v_capacitor=0 V  v_capacitor_nominal_specify=off  v_capacitor_nominal_unit=V  v_capacitor_nominal_value=1  power_dissipated_specify=off  power_dissipated_priority=None  power_dissipated=0 W  power_dissipated_nominal_specify=off  power_dissipated_nominal_unit=W  power_dissipated_nominal_value=1  thermal_network_parameterization=ee.enum.thermalNetworkTopology.cauer  Rth=[0, 10] K/W  Rth_Foster=[4, 6] K/W  thermal_mass_parameterization=ee.enum.thermalNetwork.timeconstant  thermal_mass=[0, 1] J/K  thermal_mass_Foster=[1.5, 3] J/K  thermal_time_constant=[0, 10] s  thermal_time_constant_Foster=[6, 18] s  thermal_mass_initial_temperatures=[25, 25] degC
  Diode1 : fl_lib/Electrical/Electrical Elements/Diode  Vf=0.6 V  Ron=Ron Ohm  Goff=1e-8 1/Ohm  i_specify=off  i_priority=None  i=0 A  i_nominal_specify=off  i_nominal_unit=A  i_nominal_value=1  v_specify=off  v_priority=None  v=0 V  v_nominal_specify=off  v_nominal_unit=V  v_nominal_value=1
  Switch : fl_lib/Electrical/Electrical Elements/Switch  R_closed=Ron Ohm  G_open=1e-8 1/Ohm  Threshold=0.5  i_specify=off  i_priority=None  i=0 A  i_nominal_specify=off  i_nominal_unit=A  i_nominal_value=1  v_specify=off  v_priority=None  v=0 V  v_nominal_specify=off  v_nominal_unit=V  v_nominal_value=1
  G : PMIOPort  Side=Left
  D : PMIOPort  Port=2  Side=Left
  S : PMIOPort  Port=3  Side=Right
  connections:
  G/RConn1 -- Switch/RConn1
  Switch/LConn1 -- D/RConn1 -- Diode/RConn1
  S/RConn1 -- Switch/RConn2 -- Diode/LConn1

== system pmsm_vector_ctrl_osm_2021_07_20/pmsm_simscape/AFE/SW5 ==
  Diode : ee_lib/Semiconductors & Converters/Diode  ModelType=ee.enum.diode.modelType.pwl  Vf=1.9 V  Ron=Ron Ohm  Goff=1e-8 S  prmExp=ee.enum.diode.expParam.useTwo  I12=[.0137, .545] A  V12=[.6, .7] V  IS=1e-12 A  ec=1  I1=0.0137 A  V1=0.6 V  RS=0 Ohm  Tmeas=25 degC  N_series=1  N_parallel=1  Rz=0.3 Ohm  BV=inf V  C_param=ee.enum.diode.capParam.fixed  CJ=5 pF  CJ0=5 pF  VJ=1 V  Mgrad=0.5  Vvec=[.1, 10, 100] V  Cvec=[3.5, 1, .4] pF  FC=0.5  Q_param=ee.enum.diode.recoveryParam.off  iRM=-7.15 A  iF=4 A  didt=-750 A/us  trr_factor=3  trr=115 ns  Qrr=1500 s*uA  TT=50 ns  tau=100 ns  T_param=ee.enum.diode.temperatureParam.off  IS_T2=1.25e-7 A  I1_T2=0.245 A  V1_T2=0.5 V  Tmeas2=125 degC  EG_param=ee.enum.diode.egapParam.material_si  EG=1.11 eV  XTI_param=ee.enum.diode.xtiParam.pn  XTI=3  dBVdT=0 V/K  Tdevice=25 degC  i_specify=off  i_priority=None  i=0 A  i_nominal_specify=off  i_nominal_unit=A  i_nominal_value=1  v_specify=off  v_priority=None  v=0 V  v_nominal_specify=off  v_nominal_unit=V  v_nominal_value=1  i_capacitor_specify=off  i_capacitor_priority=None  i_capacitor=0 A  i_capacitor_nominal_specify=off  i_capacitor_nominal_unit=A  i_capacitor_nominal_value=1  v_capacitor_specify=off  v_capacitor_priority=None  v_capacitor=0 V  v_capacitor_nominal_specify=off  v_capacitor_nominal_unit=V  v_capacitor_nominal_value=1  power_dissipated_specify=off  power_dissipated_priority=None  power_dissipated=0 W  power_dissipated_nominal_specify=off  power_dissipated_nominal_unit=W  power_dissipated_nominal_value=1  thermal_network_parameterization=ee.enum.thermalNetworkTopology.cauer  Rth=[0, 10] K/W  Rth_Foster=[4, 6] K/W  thermal_mass_parameterization=ee.enum.thermalNetwork.timeconstant  thermal_mass=[0, 1] J/K  thermal_mass_Foster=[1.5, 3] J/K  thermal_time_constant=[0, 10] s  thermal_time_constant_Foster=[6, 18] s  thermal_mass_initial_temperatures=[25, 25] degC
  Diode1 : fl_lib/Electrical/Electrical Elements/Diode  Vf=0.6 V  Ron=Ron Ohm  Goff=1e-8 1/Ohm  i_specify=off  i_priority=None  i=0 A  i_nominal_specify=off  i_nominal_unit=A  i_nominal_value=1  v_specify=off  v_priority=None  v=0 V  v_nominal_specify=off  v_nominal_unit=V  v_nominal_value=1
  Switch : fl_lib/Electrical/Electrical Elements/Switch  R_closed=Ron Ohm  G_open=1e-8 1/Ohm  Threshold=0.5  i_specify=off  i_priority=None  i=0 A  i_nominal_specify=off  i_nominal_unit=A  i_nominal_value=1  v_specify=off  v_priority=None  v=0 V  v_nominal_specify=off  v_nominal_unit=V  v_nominal_value=1
  G : PMIOPort  Side=Left
  D : PMIOPort  Port=2  Side=Left
  S : PMIOPort  Port=3  Side=Right
  connections:
  Diode/LConn1 -- Switch/RConn2 -- S/RConn1
  Diode/RConn1 -- D/RConn1 -- Switch/LConn1
  G/RConn1 -- Switch/RConn1

== system pmsm_vector_ctrl_osm_2021_07_20/pmsm_simscape/AFE/SW6 ==
  Diode : ee_lib/Semiconductors & Converters/Diode  ModelType=ee.enum.diode.modelType.pwl  Vf=1.9 V  Ron=Ron Ohm  Goff=1e-8 S  prmExp=ee.enum.diode.expParam.useTwo  I12=[.0137, .545] A  V12=[.6, .7] V  IS=1e-12 A  ec=1  I1=0.0137 A  V1=0.6 V  RS=0 Ohm  Tmeas=25 degC  N_series=1  N_parallel=1  Rz=0.3 Ohm  BV=inf V  C_param=ee.enum.diode.capParam.fixed  CJ=5 pF  CJ0=5 pF  VJ=1 V  Mgrad=0.5  Vvec=[.1, 10, 100] V  Cvec=[3.5, 1, .4] pF  FC=0.5  Q_param=ee.enum.diode.recoveryParam.off  iRM=-7.15 A  iF=4 A  didt=-750 A/us  trr_factor=3  trr=115 ns  Qrr=1500 s*uA  TT=50 ns  tau=100 ns  T_param=ee.enum.diode.temperatureParam.off  IS_T2=1.25e-7 A  I1_T2=0.245 A  V1_T2=0.5 V  Tmeas2=125 degC  EG_param=ee.enum.diode.egapParam.material_si  EG=1.11 eV  XTI_param=ee.enum.diode.xtiParam.pn  XTI=3  dBVdT=0 V/K  Tdevice=25 degC  i_specify=off  i_priority=None  i=0 A  i_nominal_specify=off  i_nominal_unit=A  i_nominal_value=1  v_specify=off  v_priority=None  v=0 V  v_nominal_specify=off  v_nominal_unit=V  v_nominal_value=1  i_capacitor_specify=off  i_capacitor_priority=None  i_capacitor=0 A  i_capacitor_nominal_specify=off  i_capacitor_nominal_unit=A  i_capacitor_nominal_value=1  v_capacitor_specify=off  v_capacitor_priority=None  v_capacitor=0 V  v_capacitor_nominal_specify=off  v_capacitor_nominal_unit=V  v_capacitor_nominal_value=1  power_dissipated_specify=off  power_dissipated_priority=None  power_dissipated=0 W  power_dissipated_nominal_specify=off  power_dissipated_nominal_unit=W  power_dissipated_nominal_value=1  thermal_network_parameterization=ee.enum.thermalNetworkTopology.cauer  Rth=[0, 10] K/W  Rth_Foster=[4, 6] K/W  thermal_mass_parameterization=ee.enum.thermalNetwork.timeconstant  thermal_mass=[0, 1] J/K  thermal_mass_Foster=[1.5, 3] J/K  thermal_time_constant=[0, 10] s  thermal_time_constant_Foster=[6, 18] s  thermal_mass_initial_temperatures=[25, 25] degC
  Diode1 : fl_lib/Electrical/Electrical Elements/Diode  Vf=0.6 V  Ron=Ron Ohm  Goff=1e-8 1/Ohm  i_specify=off  i_priority=None  i=0 A  i_nominal_specify=off  i_nominal_unit=A  i_nominal_value=1  v_specify=off  v_priority=None  v=0 V  v_nominal_specify=off  v_nominal_unit=V  v_nominal_value=1
  Switch : fl_lib/Electrical/Electrical Elements/Switch  R_closed=Ron Ohm  G_open=1e-8 1/Ohm  Threshold=0.5  i_specify=off  i_priority=None  i=0 A  i_nominal_specify=off  i_nominal_unit=A  i_nominal_value=1  v_specify=off  v_priority=None  v=0 V  v_nominal_specify=off  v_nominal_unit=V  v_nominal_value=1
  G : PMIOPort  Side=Left
  D : PMIOPort  Port=2  Side=Left
  S : PMIOPort  Port=3  Side=Right
  connections:
  G/RConn1 -- Switch/RConn1
  Switch/LConn1 -- D/RConn1 -- Diode/RConn1
  S/RConn1 -- Switch/RConn2 -- Diode/LConn1

== system pmsm_vector_ctrl_osm_2021_07_20/pmsm_simscape/INVERTER Control/PWM generator1 ==
  uab : Inport
  Constant : Constant  Value=0
  Constant1 : Constant
  Divide : Product  Inputs=*/
  Divide1 : Product  Inputs=*/
  PWM new cm modulation : Subsystem
  Saturation : Saturate  UpperLimit=inf  LowerLimit=eps
  m : Outport
  wires:
  uab/1 -> Divide/1
  Constant1/1 -> Saturation/1
  PWM new cm modulation/1(PWMout) -> m/1
  Divide/1 -> PWM new cm modulation/1(ab)
  Saturation/1 -> Divide1/2, Divide/2
  Divide1/1 -> PWM new cm modulation/2(m_cm)
  Constant/1 -> Divide1/1

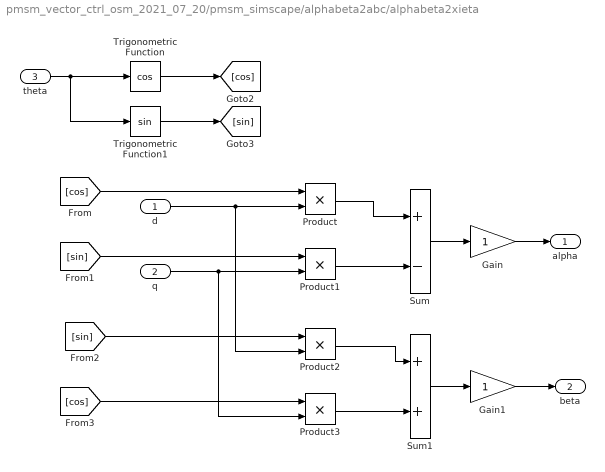
== system pmsm_vector_ctrl_osm_2021_07_20/pmsm_simscape/alphabeta2abc/alphabeta2xieta ==
  d : Inport
  q : Inport  Port=2
  theta : Inport  Port=3
  Gain : Gain
  Gain1 : Gain
  Product{,1..3} (4 alike) : Product  RndMeth=Zero
  Sum : Sum  Inputs=+-
  Sum1 : Sum
  Trigonometric Function : Trigonometry  Operator=cos
  Trigonometric Function1 : Trigonometry
  alpha : Outport  VectorParamsAs1DForOutWhenUnconnected=off
  beta : Outport  Port=2  VectorParamsAs1DForOutWhenUnconnected=off
  wires:
  theta/1 -> Trigonometric Function1/1, Trigonometric Function/1
  Trigonometric Function/1 -> [cos]
  Trigonometric Function1/1 -> [sin]
  Gain1/1 -> beta/1
  Gain/1 -> alpha/1
  Sum1/1 -> Gain1/1
  [cos] -> Product3/1
  Product3/1 -> Sum1/2
  Product2/1 -> Sum1/1
  [sin] -> Product2/1
  Sum/1 -> Gain/1
  q/1 -> Product1/2, Product3/2
  [sin] -> Product1/1
  Product1/1 -> Sum/2
  Product/1 -> Sum/1
  d/1 -> Product2/2, Product/2
  [cos] -> Product/1
